simulink model "Untitled1"  (R2013b)
settings: Solver=ode4  StartTime=0.0  StopTime=tSim  FixedStep=h  RelTol=1e-3
values from neighbouring files (symbols this model uses):
  k = zeros(7,1)    [dp.m]    (also in launcher.m = 200)
  w = 1    [launcher.m]    (also in launcher2.m = [t;sin(t)]')
  y0 = 0    [launcher.m]    (also in launcher2.m = 1)
settings Model: Creator=JAR  LastModifiedBy=JAR

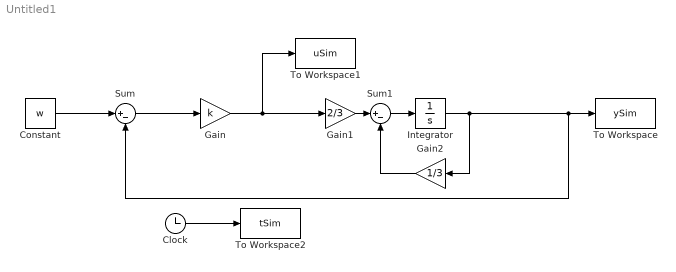
== system Untitled1 ==
  Clock : Clock
  Constant : Constant  Value=w
  Gain : Gain  Gain=k
  Gain1 : Gain  Gain=2/3
  Gain2 : Gain  Gain=1/3
  Integrator : Integrator  InitialCondition=y0
  Sum : Sum  Inputs=|+-
  Sum1 : Sum  Inputs=|+-
  To Workspace : ToWorkspace  VariableName=ySim  SampleTime=-1
  To Workspace1 : ToWorkspace  VariableName=uSim  SampleTime=-1
  To Workspace2 : ToWorkspace  VariableName=tSim  SampleTime=-1
  wires:
  Sum/1 -> Gain/1
  Constant/1 -> Sum/1
  Clock/1 -> To Workspace2/1
  Gain1/1 -> Sum1/1
  Gain2/1 -> Sum1/2
  Sum1/1 -> Integrator/1
  Integrator/1 -> Sum/2, To Workspace/1, Gain2/1
  Gain/1 -> To Workspace1/1, Gain1/1
